simulink model "sistema_final_2018a"  (R2018a)
settings: Solver=FixedStepAuto  StartTime=0.0  StopTime=2000  FixedStep=0.01  RelTol=1e-3
undefined symbols (not defined in the file or in its folder): serial
libraries: simulink x6, instrumentlib x3, imaqlib x2
settings Model: PauseTimes=10  Creator=eduardo  LastModifiedBy=eduardo
settings DebuggingCC: LibraryContextMissingDiagnostic=warning
settings SFSimCC: SimUseLocalCustomCode=on
settings RTWCC: RTWUseLocalCustomCode=on

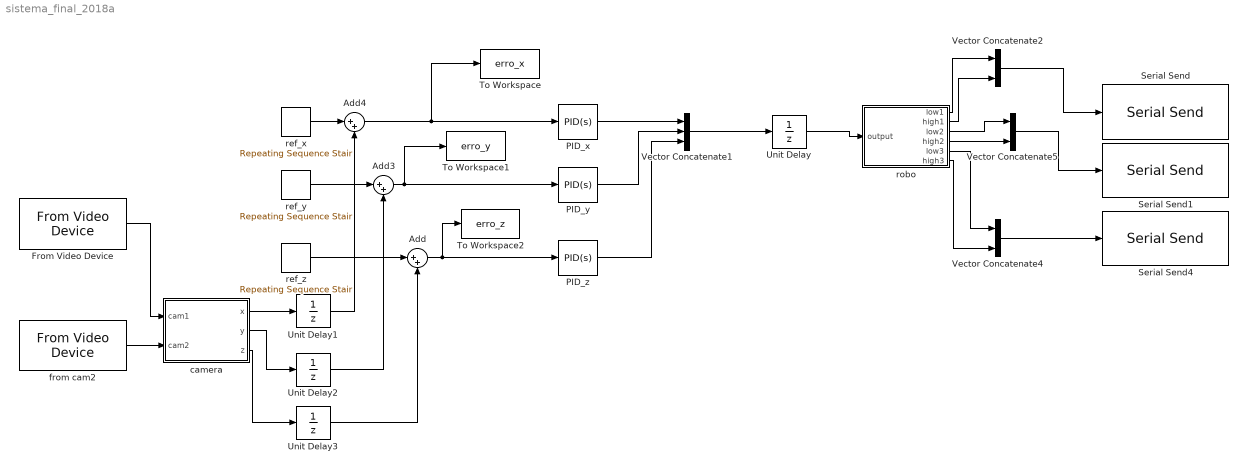
== system sistema_final_2018a ==
  Add : Sum  Inputs=|++
  Add3 : Sum  Inputs=|++
  Add4 : Sum  Inputs=|++
  From Video Device : imaqlib/From Video Device  DeviceMenu=(none)  Device=winvideo 1 (Logitech HD Webcam C270)  ObjConstructor=(none)  VideoFormatMenu=(none)  VideoFormat=(none)  VideoSource=none  ROIPosition=[0 0 480 640]  EnableHWTrigger=off  TriggerConfiguration=winvideo 1 (Logitech HD Webcam C270)  SampleTime=0.01  OutputPortsMode=One multidimensional signal  DataType=uint32  CanDoHWTrigger=no  ReturnedColorSpace=rgb  BlockHandle=8939.0001  ROIWidth=640  ROIHeight=480  ROIColumn=0  ROIRow=0  EngXMLPath=C:\Program Files\MATLAB\R2018b\toolbox\imaq\imaq\private  DevXMLPath=C:\ProgramData\MATLAB\SupportPackages\R2018b\toolbox\imaq\supportpackages\genericvideo\adaptor\win64  EngLibPath=C:\Program Files\MATLAB\R2018b\toolbox\imaq\imaqblks\imaqmex\win64  ColorSpace=rgb  BayerSensorAlignment=grbg
      settings: SourceProductName=Image Acquisition Toolbox
  PID_x : simulink/Continuous/PID Controller  Controller=PID  Form=Parallel  TimeDomain=Continuous-time  SampleTime=-1  IntegratorMethod=Forward Euler  FilterMethod=Forward Euler  ControllerParametersSource=internal  P=124.231  I=164.8199  D=-380.1082  UseFilter=on  N=100  TunerSelectOption=Transfer Function Based (PID Tuner App)  InitialConditionSource=internal  InitialConditionForIntegrator=0  InitialConditionForFilter=0  DifferentiatorICPrevScaledInput=0  ExternalReset=none  TrackingMode=off  Kt=1  LimitOutput=off  UpperSaturationLimit=inf  LowerSaturationLimit=-inf  LinearizeAsGain=on  AntiWindupMode=none  Kb=1  POutMin=[]  POutMax=[]  IOutMin=[]  IOutMax=[]  DOutMin=[]  DOutMax=[]  NOutMin=[]  NOutMax=[]  SumOutMin=[]  SumOutMax=[]  SaturationOutMin=[]  SaturationOutMax=[]  PParamMin=[]  PParamMax=[]  IParamMin=[]  IParamMax=[]  DParamMin=[]  DParamMax=[]  NParamMin=[]  NParamMax=[]  KbParamMin=[]  KbParamMax=[]  KtParamMin=[]  KtParamMax=[]  KbOutMin=[]  KbOutMax=[]  KtOutMin=[]  KtOutMax=[]  IntegratorOutMin=[]  IntegratorOutMax=[]  FilterOutMin=[]  FilterOutMax=[]  SumI1OutMin=[]  SumI1OutMax=[]  SumI2OutMin=[]  SumI2OutMax=[]  SumI3OutMin=[]  SumI3OutMax=[]  SumDOutMin=[]  SumDOutMax=[]  DifferentiatorOutMin=[]  DifferentiatorOutMax=[]  FilterDiffOutCoefMin=[]  FilterDiffOutCoefMax=[]  ReciprocalOutMin=[]  ReciprocalOutMax=[]  SumDenOutMin=[]  SumDenOutMax=[]  SumNumOutMin=[]  SumNumOutMax=[]  DivideOutMin=[]  DivideOutMax=[]  IntegratorContinuousStateAttributes=''  IntegratorStateMustResolveToSignalObject=off  IntegratorRTWStateStorageClass=Auto  FilterContinuousStateAttributes=''  FilterStateMustResolveToSignalObject=off  FilterRTWStateStorageClass=Auto
  PID_y : simulink/Continuous/PID Controller  Controller=PID  Form=Parallel  TimeDomain=Continuous-time  SampleTime=-1  IntegratorMethod=Forward Euler  FilterMethod=Forward Euler  ControllerParametersSource=internal  P=1335.7759  I=763.3354  D=431.593  UseFilter=on  N=100  TunerSelectOption=Transfer Function Based (PID Tuner App)  InitialConditionSource=internal  InitialConditionForIntegrator=0  InitialConditionForFilter=0  DifferentiatorICPrevScaledInput=0  ExternalReset=none  TrackingMode=off  Kt=1  LimitOutput=off  UpperSaturationLimit=inf  LowerSaturationLimit=-inf  LinearizeAsGain=on  AntiWindupMode=none  Kb=1  POutMin=[]  POutMax=[]  IOutMin=[]  IOutMax=[]  DOutMin=[]  DOutMax=[]  NOutMin=[]  NOutMax=[]  SumOutMin=[]  SumOutMax=[]  SaturationOutMin=[]  SaturationOutMax=[]  PParamMin=[]  PParamMax=[]  IParamMin=[]  IParamMax=[]  DParamMin=[]  DParamMax=[]  NParamMin=[]  NParamMax=[]  KbParamMin=[]  KbParamMax=[]  KtParamMin=[]  KtParamMax=[]  KbOutMin=[]  KbOutMax=[]  KtOutMin=[]  KtOutMax=[]  IntegratorOutMin=[]  IntegratorOutMax=[]  FilterOutMin=[]  FilterOutMax=[]  SumI1OutMin=[]  SumI1OutMax=[]  SumI2OutMin=[]  SumI2OutMax=[]  SumI3OutMin=[]  SumI3OutMax=[]  SumDOutMin=[]  SumDOutMax=[]  DifferentiatorOutMin=[]  DifferentiatorOutMax=[]  FilterDiffOutCoefMin=[]  FilterDiffOutCoefMax=[]  ReciprocalOutMin=[]  ReciprocalOutMax=[]  SumDenOutMin=[]  SumDenOutMax=[]  SumNumOutMin=[]  SumNumOutMax=[]  DivideOutMin=[]  DivideOutMax=[]  IntegratorContinuousStateAttributes=''  IntegratorStateMustResolveToSignalObject=off  IntegratorRTWStateStorageClass=Auto  FilterContinuousStateAttributes=''  FilterStateMustResolveToSignalObject=off  FilterRTWStateStorageClass=Auto
  PID_z : simulink/Continuous/PID Controller  Controller=PID  Form=Parallel  TimeDomain=Continuous-time  SampleTime=-1  IntegratorMethod=Forward Euler  FilterMethod=Forward Euler  ControllerParametersSource=internal  P=113.7205  I=315.8587  D=-342.2963  UseFilter=on  N=100  TunerSelectOption=Transfer Function Based (PID Tuner App)  InitialConditionSource=internal  InitialConditionForIntegrator=0  InitialConditionForFilter=0  DifferentiatorICPrevScaledInput=0  ExternalReset=none  TrackingMode=off  Kt=1  LimitOutput=off  UpperSaturationLimit=inf  LowerSaturationLimit=-inf  LinearizeAsGain=on  AntiWindupMode=none  Kb=1  POutMin=[]  POutMax=[]  IOutMin=[]  IOutMax=[]  DOutMin=[]  DOutMax=[]  NOutMin=[]  NOutMax=[]  SumOutMin=[]  SumOutMax=[]  SaturationOutMin=[]  SaturationOutMax=[]  PParamMin=[]  PParamMax=[]  IParamMin=[]  IParamMax=[]  DParamMin=[]  DParamMax=[]  NParamMin=[]  NParamMax=[]  KbParamMin=[]  KbParamMax=[]  KtParamMin=[]  KtParamMax=[]  KbOutMin=[]  KbOutMax=[]  KtOutMin=[]  KtOutMax=[]  IntegratorOutMin=[]  IntegratorOutMax=[]  FilterOutMin=[]  FilterOutMax=[]  SumI1OutMin=[]  SumI1OutMax=[]  SumI2OutMin=[]  SumI2OutMax=[]  SumI3OutMin=[]  SumI3OutMax=[]  SumDOutMin=[]  SumDOutMax=[]  DifferentiatorOutMin=[]  DifferentiatorOutMax=[]  FilterDiffOutCoefMin=[]  FilterDiffOutCoefMax=[]  ReciprocalOutMin=[]  ReciprocalOutMax=[]  SumDenOutMin=[]  SumDenOutMax=[]  SumNumOutMin=[]  SumNumOutMax=[]  DivideOutMin=[]  DivideOutMax=[]  IntegratorContinuousStateAttributes=''  IntegratorStateMustResolveToSignalObject=off  IntegratorRTWStateStorageClass=Auto  FilterContinuousStateAttributes=''  FilterStateMustResolveToSignalObject=off  FilterRTWStateStorageClass=Auto
  Serial Send : instrumentlib/Serial Send  ComPortMenu=<Please select a port...>  ComPort=COM3  ObjConstructor=serial('COM3');  Terminator=<none>  EnableBlockingMode=on
  Serial Send1 : instrumentlib/Serial Send  ComPortMenu=<Please select a port...>  ComPort=COM3  ObjConstructor=serial('COM3');  Terminator=<none>  EnableBlockingMode=on
  Serial Send4 : instrumentlib/Serial Send  ComPortMenu=<Please select a port...>  ComPort=COM3  ObjConstructor=serial('COM3');  Terminator=<none>  EnableBlockingMode=on
  To Workspace : ToWorkspace  VariableName=erro_x  SampleTime=-1
  To Workspace1 : ToWorkspace  VariableName=erro_y  SampleTime=-1
  To Workspace2 : ToWorkspace  VariableName=erro_z  SampleTime=-1
  Unit Delay{,1..3} (4 alike) : UnitDelay  SampleTime=-1
  Vector Concatenate1 : Concatenate  NumInputs=3
  Vector Concatenate2 : Concatenate
  Vector Concatenate4 : Concatenate
  Vector Concatenate5 : Concatenate
  camera : MATLAB Function  TreatAsAtomicUnit=on
  "from cam2 " : imaqlib/From Video Device  DeviceMenu=(none)  Device=winvideo 2 (Logitech HD Webcam C270)  ObjConstructor=(none)  VideoFormatMenu=(none)  VideoFormat=(none)  VideoSource=none  ROIPosition=[0 0 480 640]  EnableHWTrigger=off  TriggerConfiguration=winvideo 1 (Logitech HD Webcam C270)  SampleTime=0.01  OutputPortsMode=One multidimensional signal  DataType=uint32  CanDoHWTrigger=no  ReturnedColorSpace=rgb  BlockHandle=8939.0001  ROIWidth=640  ROIHeight=480  ROIColumn=0  ROIRow=0  EngXMLPath=C:\Program Files\MATLAB\R2018b\toolbox\imaq\imaq\private  DevXMLPath=C:\ProgramData\MATLAB\SupportPackages\R2018b\toolbox\imaq\supportpackages\genericvideo\adaptor\win64  EngLibPath=C:\Program Files\MATLAB\R2018b\toolbox\imaq\imaqblks\imaqmex\win64  ColorSpace=rgb  BayerSensorAlignment=grbg
      settings: SourceProductName=Image Acquisition Toolbox
  ref_x : simulink/Sources/Repeating Sequence Stair  OutValues=ref_x  tsamp=1  OutMin=[]  OutMax=[]  OutDataTypeStr=double  OutputDataTypeScalingMode=double  OutDataType=fixdt(0,8)  ConRadixGroup=Best Precision: Vector-wise  OutScaling=2^-12
  ref_y : simulink/Sources/Repeating Sequence Stair  OutValues=ref_y  tsamp=1  OutMin=[]  OutMax=[]  OutDataTypeStr=double  OutputDataTypeScalingMode=double  OutDataType=fixdt(0,8)  ConRadixGroup=Best Precision: Vector-wise  OutScaling=2^-12
  ref_z : simulink/Sources/Repeating Sequence Stair  OutValues=ref_z  tsamp=1  OutMin=[]  OutMax=[]  OutDataTypeStr=double  OutputDataTypeScalingMode=double  OutDataType=fixdt(0,8)  ConRadixGroup=Best Precision: Vector-wise  OutScaling=2^-12
  robo : MATLAB Function  TreatAsAtomicUnit=on
  wires:
  PID_z/1 -> Vector Concatenate1/3
  ref_z/1 -> Add/1
  ref_x/1 -> Add4/1
  ref_y/1 -> Add3/1
  Add4/1 -> To Workspace/1, PID_x/1
  PID_x/1 -> Vector Concatenate1/1
  PID_y/1 -> Vector Concatenate1/2
  Vector Concatenate1/1 -> Unit Delay/1
  Unit Delay/1 -> robo/1(output)
  Add3/1 -> To Workspace1/1, PID_y/1
  Add/1 -> To Workspace2/1, PID_z/1
  robo/1(low1) -> Vector Concatenate2/1
  robo/2(high1) -> Vector Concatenate2/2
  Vector Concatenate2/1 -> Serial Send/1
  robo/3(low2) -> Vector Concatenate5/1
  robo/4(high2) -> Vector Concatenate5/2
  robo/6(high3) -> Vector Concatenate4/2
  robo/5(low3) -> Vector Concatenate4/1
  Vector Concatenate5/1 -> Serial Send1/1
  Vector Concatenate4/1 -> Serial Send4/1
  camera/1(x) -> Unit Delay1/1
  camera/2(y) -> Unit Delay2/1
  camera/3(z) -> Unit Delay3/1
  From Video Device/1 -> camera/1(cam1)
  "from cam2 "/1 -> camera/2(cam2)
  Unit Delay1/1 -> Add4/2
  Unit Delay2/1 -> Add3/2
  Unit Delay3/1 -> Add/2

== matlab function sistema_final_2018a/camera ==
  data: x output; y output; z output; cam1 input; cam2 input
function [x,y,z]  = camera(cam1, cam2)
success=0;
data = load('amarelo.mat', 'LAB');
LAB = data.LAB;
pos=[1,1,1]; 
while success==0
   stat1 = detectLABColor(cam1, LAB);
   stat2 = detectLABColor(cam2, LAB);
   % [pos,success] = triangular(stat1, stat2, stereoParams);  
   pos=[1,1,1]; 
   success=1; 
end
x=pos(1);
y=pos(2);
z=pos(3);

end

== matlab function sistema_final_2018a/robo ==
  data: low1 output; output input; high1 output; low2 output; high2 output; low3 output; high3 output
function [low1,high1,low2,high2,low3,high3] = robo(output)

s2 = output(1);
s3 = output(2);
s4 = output(3);
low1 = mod (s2, 256);
high1 = floor(s2/256);
low2 = mod (s3, 256);
high2 = floor(s3/256);
low3 = mod (s4, 256);
high3 = floor(s4/256);

end
